simulink subsystem "SurfEngRef"  (R2025a)
settings: Solver=VariableStepAuto  StartTime=0.0  StopTime=10.0  RelTol=1e-3
undefined symbols (not defined in the file): SimIn, SimPar
libraries: simulink x42, ServosLib x6
(part 1 of 2)
settings Model: Creator=drhill  LastModifiedBy=alhallmark
settings SolverCC: AlgebraicLoopSolver=TrustRegion
settings OptimizationCC: ReuseModelBlockBuffer=off
settings DebuggingCC: UnconnectedInputMsg=warning  UnconnectedOutputMsg=warning  UnconnectedLineMsg=warning
settings ModelReferenceCC: EnableRefExpFcnMdlSchedulingChecks=on
settings RTWCC: GPUComputeCapability=3.5  DLArmComputeVersion=19.05

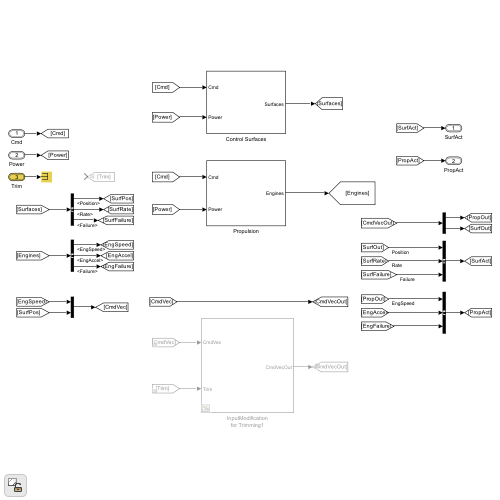
[thumbnail: Simulink's stored preview of the top-level diagram]
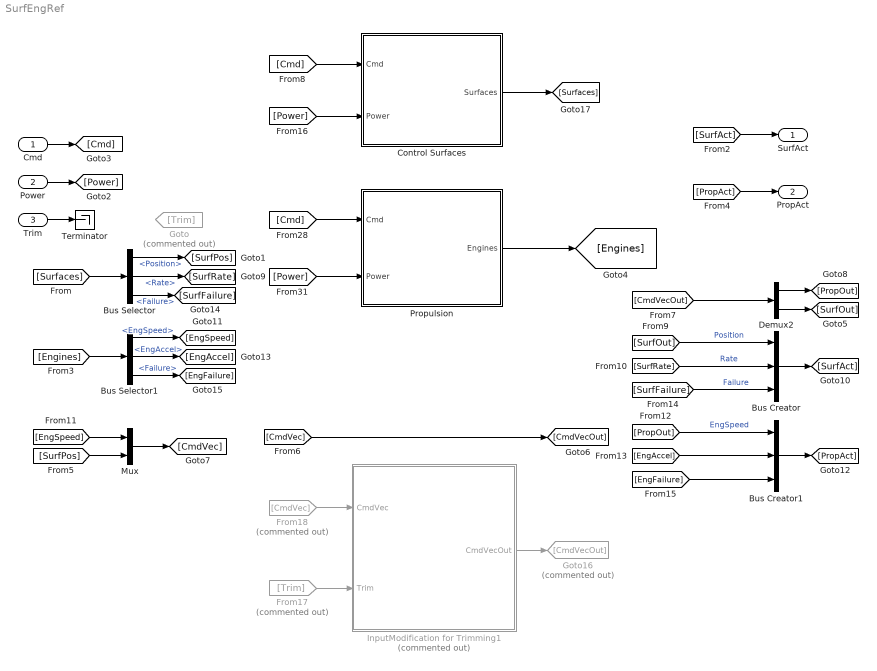
== system SurfEngRef ==
  Cmd : Inport  OutDataTypeStr=Bus: BUS_CMD
  Power : Inport  Port=2  OutDataTypeStr=Bus: BUS_POWER_SYSTEM_OUT
  Trim : Inport  Port=3  OutDataTypeStr=Bus: BUS_TRIM_INPUT
  Bus Creator : BusCreator  Inputs=3  OutDataTypeStr=Bus: BUS_SURF_ACTUATOR
  Bus Creator1 : BusCreator  Inputs=3  OutDataTypeStr=Bus: BUS_PROP_ACTUATOR
  Bus Selector : BusSelector  OutputSignals=Position,Rate,Failure
  Bus Selector1 : BusSelector  OutputSignals=EngSpeed,EngAccel,Failure
  Control Surfaces : Subsystem  VariantControl=GVS_ACT_TYPE_NONE
  Demux2 : Demux  Outputs=[SimIn.numEngines SimIn.numSurfaces]
  From17 : From  Commented=on  GotoTag=Trim
  From18 : From  Commented=on  GotoTag=CmdVec
  Goto : Goto  Commented=on  GotoTag=Trim
  Goto16 : Goto  Commented=on  GotoTag=CmdVecOut
  InputModification for Trimming1 : Subsystem  Commented=on
  Mux : Mux  Inputs=[SimIn.numEngines SimIn.numSurfaces]
  Propulsion : Subsystem  VariantControl=GVS_PROP_TYPE_NONE
  Terminator : Terminator
  SurfAct : Outport  OutDataTypeStr=Bus: BUS_SURF_ACTUATOR
  PropAct : Outport  Port=2  OutDataTypeStr=Bus: BUS_PROP_ACTUATOR
  wires:
  [Cmd] -> Control Surfaces/1(Cmd)
  [Power] -> Control Surfaces/2(Power)
  Control Surfaces/1(Surfaces) -> [Surfaces]
  Trim/1 -> Terminator/1
  Power/1 -> [Power]
  Cmd/1 -> [Cmd]
  [SurfAct] -> SurfAct/1
  [Power] -> Propulsion/2(Power)
  Propulsion/1(Engines) -> [Engines]
  [PropAct] -> PropAct/1
  [Cmd] -> Propulsion/1(Cmd)
  [CmdVec] -> [CmdVecOut]
  Mux/1 -> [CmdVec]
  [CmdVecOut] -> Demux2/1
  Demux2/2 -> [SurfOut]
  Demux2/1 -> [PropOut]
  [Surfaces] -> Bus Selector/1
  Bus Selector/1 -> [SurfPos]  "<Position>"
  [SurfPos] -> Mux/2
  [SurfOut] -> Bus Creator/1  "Position"
  Bus Selector/2 -> [SurfRate]  "<Rate>"
  [SurfRate] -> Bus Creator/2  "Rate"
  Bus Creator/1 -> [SurfAct]
  [Engines] -> Bus Selector1/1
  Bus Selector1/1 -> [EngSpeed]  "<EngSpeed>"
  [EngSpeed] -> Mux/1
  [PropOut] -> Bus Creator1/1  "EngSpeed"
  Bus Creator1/1 -> [PropAct]
  Bus Selector1/2 -> [EngAccel]  "<EngAccel>"
  [EngAccel] -> Bus Creator1/2
  Bus Selector/3 -> [SurfFailure]  "<Failure>"
  [SurfFailure] -> Bus Creator/3  "Failure"
  Bus Selector1/3 -> [EngFailure]  "<Failure>"
  [EngFailure] -> Bus Creator1/3
  InputModification for Trimming1/1(CmdVecOut) -> Goto16/1
  From18/1 -> InputModification for Trimming1/1(CmdVec)
  From17/1 -> InputModification for Trimming1/2(Trim)

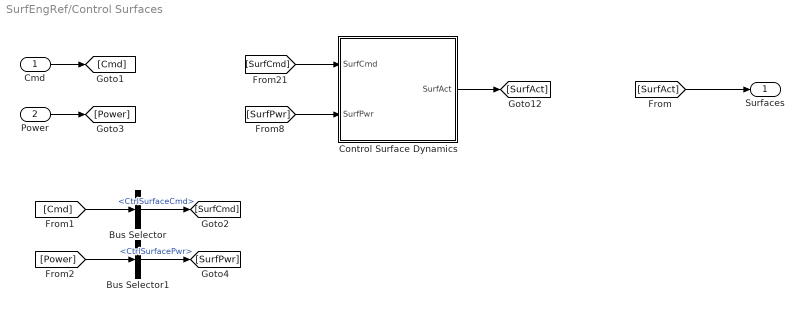
== system SurfEngRef/Control Surfaces ==
  Cmd : Inport
  Power : Inport  Port=2
  Bus Selector : BusSelector  OutputSignals=CtrlSurfaceCmd
  Bus Selector1 : BusSelector  OutputSignals=CtrlSurfacePwr
  Control Surface Dynamics : Subsystem  Variant=on
  Surfaces : Outport  VectorParamsAs1DForOutWhenUnconnected=off
  wires:
  [Cmd] -> Bus Selector/1
  Bus Selector/1 -> [SurfCmd]  "<CtrlSurfaceCmd>"
  Bus Selector1/1 -> [SurfPwr]  "<CtrlSurfacePwr>"
  [Power] -> Bus Selector1/1
  [SurfPwr] -> Control Surface Dynamics/2(SurfPwr)
  Control Surface Dynamics/1(SurfAct) -> [SurfAct]
  [SurfCmd] -> Control Surface Dynamics/1(SurfCmd)
  Power/1 -> [Power]
  [SurfAct] -> Surfaces/1
  Cmd/1 -> [Cmd]

== system SurfEngRef/InputModification for Trimming1 ==
  CmdVec : Inport
  Trim : Inport  Port=2  OutDataTypeStr=Bus: BUS_TRIM_INPUT
  Constant : Constant  Value=SimIn.Switches.TrimModeOn
  "Invalid, Error Out" : Subsystem  TreatAsAtomicUnit=on
  Merge : Merge  Inputs=3  InitialOutput=zeros(SimIn.numEngines+SimIn.numSurfaces,1)
  SimMode:PassThrough : Subsystem  TreatAsAtomicUnit=on
  Switch Case : SwitchCase  CaseConditions={0,1}
  TrimMode: DriveFromTopLevel : Subsystem  TreatAsAtomicUnit=on
  CmdVecOut : Outport  VectorParamsAs1DForOutWhenUnconnected=off
  wires:
  [Trim] -> TrimMode: DriveFromTopLevel/1(TrimBias)
  [CmdVec] -> SimMode:PassThrough/1(Cmd)
  Trim/1 -> [Trim]
  CmdVec/1 -> [CmdVec]
  Switch Case/1 -> SimMode:PassThrough/Action
  Switch Case/2 -> TrimMode: DriveFromTopLevel/Action
  SimMode:PassThrough/1(Out) -> Merge/1
  TrimMode: DriveFromTopLevel/1(Out) -> Merge/2
  Merge/1 -> CmdVecOut/1
  Constant/1 -> Switch Case/1
  Switch Case/3 -> "Invalid, Error Out"/Action
  "Invalid, Error Out"/1(Out) -> Merge/3

== system SurfEngRef/Propulsion ==
  Cmd : Inport  OutDataTypeStr=Bus: BUS_CMD
  Power : Inport  Port=2
  Bus Selector : BusSelector  OutputSignals=EngineCmd
  Bus Selector1 : BusSelector  OutputSignals=EnginePwr
  Propulsion Dynamics : Subsystem  Variant=on
  Engines : Outport  OutDataTypeStr=Bus: BUS_PROP_ACTUATOR  VectorParamsAs1DForOutWhenUnconnected=off
  wires:
  Bus Selector1/1 -> [EngPwr]  "<EnginePwr>"
  [Power] -> Bus Selector1/1
  Bus Selector/1 -> [EngCmd]  "<EngineCmd>"
  [Cmd] -> Bus Selector/1
  [EngPwr] -> Propulsion Dynamics/2(EngPwr)
  [EngCmd] -> Propulsion Dynamics/1(EngCmd)
  Propulsion Dynamics/1(PropAct) -> [PropAct]
  [PropAct] -> Engines/1
  Power/1 -> [Power]
  Cmd/1 -> [Cmd]

== system SurfEngRef/Control Surfaces/Control Surface Dynamics ==
  SurfCmd : Inport
  SurfPwr : Inport  Port=2
  FirstOrder : Subsystem  VariantControl=GVS_ACT_TYPE_FIRSTORDER
  FirstOrderFailSurf : Subsystem  VariantControl=GVS_ACT_TYPE_FIRSTORDERFAILSURF
  None : Subsystem  VariantControl=GVS_ACT_TYPE_NONE
  SecondOrder : Subsystem  VariantControl=GVS_ACT_TYPE_SECONDORDER
  SurfAct : Outport

== system SurfEngRef/InputModification for Trimming1/Invalid, Error Out ==
  Action Port : ActionPort
  Constant1 : Constant  Value=zeros(SimIn.numEngines+SimIn.numSurfaces,1)
  Constant2 : Constant  Value=0
  InvalidMode : Assertion  AssertionFailFcn="warndlg('Invalid settings for TrimMode and LinearizeMode.  Run setup.m to reset.','Warning!')"
  Out : Outport  InitialOutput=zeros(SimIn.numEngines+SimIn.numSurfaces,1)  VectorParamsAs1DForOutWhenUnconnected=off
  wires:
  Constant2/1 -> InvalidMode/1
  Constant1/1 -> Out/1

== system SurfEngRef/InputModification for Trimming1/SimMode:PassThrough ==
  Cmd : Inport
  Action Port : ActionPort
  Gain1 : Gain
  Out : Outport  InitialOutput=zeros(SimIn.numEngines+SimIn.numSurfaces,1)  VectorParamsAs1DForOutWhenUnconnected=off
  wires:
  Cmd/1 -> Gain1/1  "LiftEngines(8),TailEngine,Aileron,Flaps,Elevator,Rudder"
  Gain1/1 -> Out/1

== system SurfEngRef/InputModification for Trimming1/TrimMode: DriveFromTopLevel ==
  TrimBias : Inport  OutDataTypeStr=Bus: BUS_TRIM_INPUT
  Action Port : ActionPort
  Bus Selector : BusSelector  OutputSignals=Engines,Surfaces
  Force Consistent Sample Time on Bus : Subsystem  Commented=on
  Multiply : Gain  Gain=SimIn.Trim.surfaceAlloc  Multiplication=Matrix(K*u)
  Mux : Mux  Inputs=2
  Out : Outport  InitialOutput=zeros(SimIn.numEngines+SimIn.numSurfaces,1)  VectorParamsAs1DForOutWhenUnconnected=off
  wires:
  Mux/1 -> Out/1
  Multiply/1 -> Mux/2
  Bus Selector/1 -> Mux/1  "<Engines>"
  TrimBias/1 -> Bus Selector/1
  Bus Selector/2 -> Multiply/1  "<Surfaces>"

== system SurfEngRef/Propulsion/Propulsion Dynamics ==
  EngCmd : Inport
  EngPwr : Inport  Port=2
  FirstOrder : Subsystem  VariantControl=GVS_PROP_TYPE_FIRSTORDER
  FirstOrderFailProp : Subsystem  VariantControl=GVS_PROP_TYPE_FIRSTORDERFAILPROP
  None : Subsystem  VariantControl=GVS_PROP_TYPE_NONE
  SecondOrder : Subsystem  VariantControl=GVS_PROP_TYPE_SECONDORDER
  PropAct : Outport

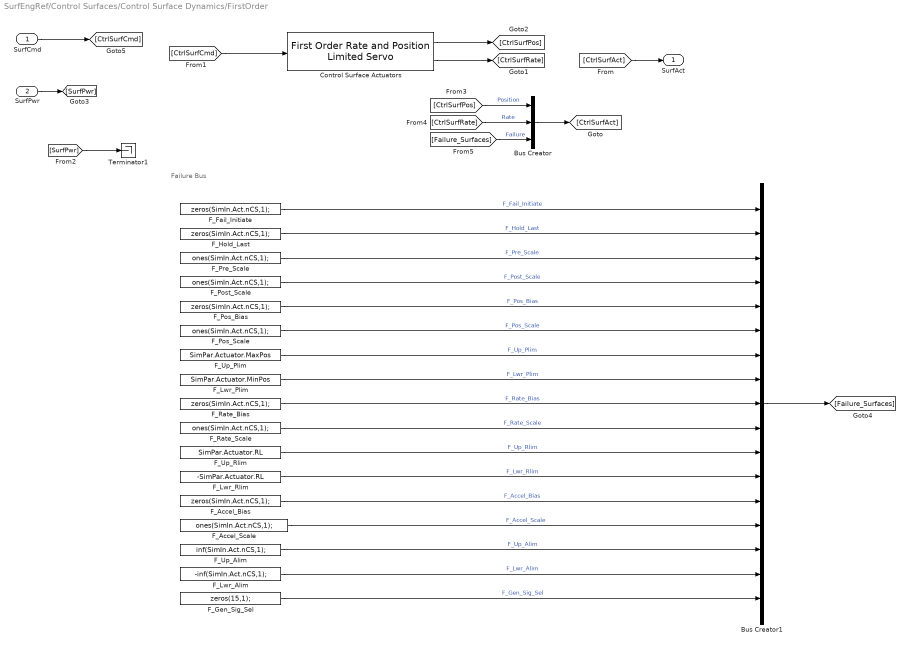
== system SurfEngRef/Control Surfaces/Control Surface Dynamics/FirstOrder ==
  note: Failure Bus
  SurfCmd : Inport
  SurfPwr : Inport  Port=2
  Bus Creator : BusCreator  Inputs=3  OutDataTypeStr=Bus: BUS_SURF_ACTUATOR
  Bus Creator1 : BusCreator  Inputs=17  OutDataTypeStr=Bus: BUS_FAILURE_SURF
  Control Surface Actuators : ServosLib/First Order  Rate and Position Limited  Servo  freq=SimPar.Actuator.BW  RL=SimPar.Actuator.RL  POS_hi=SimPar.Actuator.MaxPos  POS_lo=SimPar.Actuator.MinPos  Bias=SimPar.Actuator.Bias  StateName=Actuators
  F_Accel_Bias : Constant  Value=zeros(SimIn.Act.nCS,1);
  F_Accel_Scale : Constant  Value=ones(SimIn.Act.nCS,1);
  F_Fail_Initiate : Constant  Value=zeros(SimIn.Act.nCS,1);
  F_Gen_Sig_Sel : Constant  Value=zeros(15,1);
  F_Hold_Last : Constant  Value=zeros(SimIn.Act.nCS,1);
  F_Lwr_Alim : Constant  Value=-inf(SimIn.Act.nCS,1);
  F_Lwr_Plim : Constant  Value=SimPar.Actuator.MinPos
  F_Lwr_Rlim : Constant  Value=-SimPar.Actuator.RL
  F_Pos_Bias : Constant  Value=zeros(SimIn.Act.nCS,1);
  F_Pos_Scale : Constant  Value=ones(SimIn.Act.nCS,1);
  F_Post_Scale : Constant  Value=ones(SimIn.Act.nCS,1);
  F_Pre_Scale : Constant  Value=ones(SimIn.Act.nCS,1);
  F_Rate_Bias : Constant  Value=zeros(SimIn.Act.nCS,1);
  F_Rate_Scale : Constant  Value=ones(SimIn.Act.nCS,1);
  F_Up_Alim : Constant  Value=inf(SimIn.Act.nCS,1);
  F_Up_Plim : Constant  Value=SimPar.Actuator.MaxPos
  F_Up_Rlim : Constant  Value=SimPar.Actuator.RL
  Terminator1 : Terminator
  SurfAct : Outport
  wires:
  F_Gen_Sig_Sel/1 -> Bus Creator1/17  "F_Gen_Sig_Sel"
  F_Lwr_Alim/1 -> Bus Creator1/16  "F_Lwr_Alim"
  F_Up_Alim/1 -> Bus Creator1/15  "F_Up_Alim"
  F_Accel_Scale/1 -> Bus Creator1/14  "F_Accel_Scale"
  F_Accel_Bias/1 -> Bus Creator1/13  "F_Accel_Bias"
  F_Lwr_Rlim/1 -> Bus Creator1/12  "F_Lwr_Rlim"
  F_Up_Rlim/1 -> Bus Creator1/11  "F_Up_Rlim"
  F_Rate_Scale/1 -> Bus Creator1/10  "F_Rate_Scale"
  F_Rate_Bias/1 -> Bus Creator1/9  "F_Rate_Bias"
  F_Lwr_Plim/1 -> Bus Creator1/8  "F_Lwr_Plim"
  F_Up_Plim/1 -> Bus Creator1/7  "F_Up_Plim"
  F_Pos_Scale/1 -> Bus Creator1/6  "F_Pos_Scale"
  F_Pos_Bias/1 -> Bus Creator1/5  "F_Pos_Bias"
  F_Post_Scale/1 -> Bus Creator1/4  "F_Post_Scale"
  [Failure_Surfaces] -> Bus Creator/3  "Failure"
  F_Pre_Scale/1 -> Bus Creator1/3  "F_Pre_Scale"
  F_Hold_Last/1 -> Bus Creator1/2  "F_Hold_Last"
  Bus Creator1/1 -> [Failure_Surfaces]
  F_Fail_Initiate/1 -> Bus Creator1/1  "F_Fail_Initiate"
  [SurfPwr] -> Terminator1/1
  SurfPwr/1 -> [SurfPwr]
  SurfCmd/1 -> [CtrlSurfCmd]
  [CtrlSurfCmd] -> Control Surface Actuators/1
  Control Surface Actuators/1 -> [CtrlSurfPos]
  Control Surface Actuators/2 -> [CtrlSurfRate]
  [CtrlSurfAct] -> SurfAct/1
  [CtrlSurfPos] -> Bus Creator/1  "Position"
  [CtrlSurfRate] -> Bus Creator/2  "Rate"
  Bus Creator/1 -> [CtrlSurfAct]

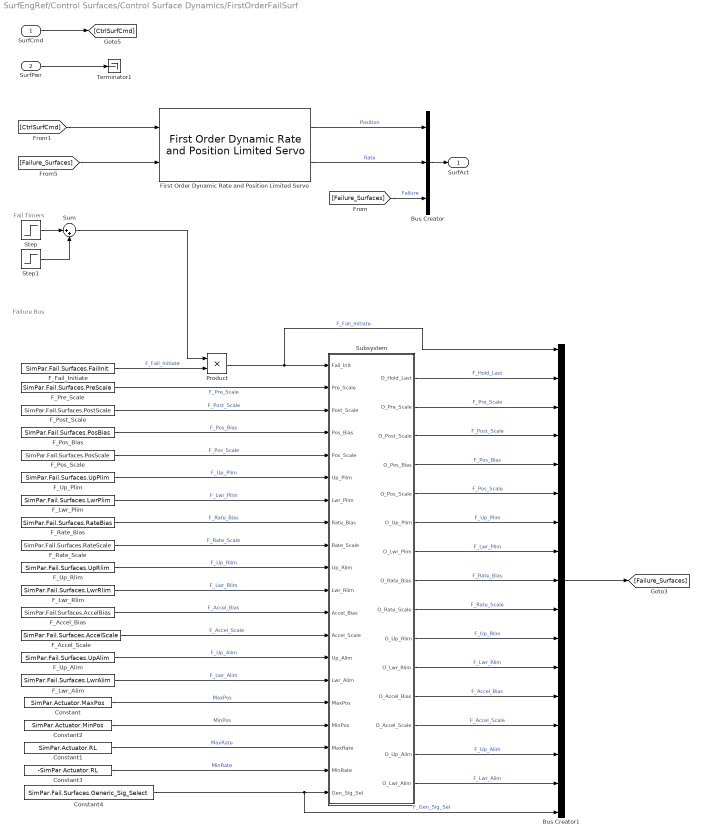
== system SurfEngRef/Control Surfaces/Control Surface Dynamics/FirstOrderFailSurf ==
  note: Failure Bus
  note: Fail Timers
  SurfCmd : Inport
  SurfPwr : Inport  Port=2
  Bus Creator : BusCreator  Inputs=3  OutDataTypeStr=Bus: BUS_SURF_ACTUATOR
  Bus Creator1 : BusCreator  Inputs=17  OutDataTypeStr=Bus: BUS_FAILURE_SURF
  Constant : Constant  Value=SimPar.Actuator.MaxPos
  Constant1 : Constant  Value=SimPar.Actuator.RL
  Constant2 : Constant  Value=SimPar.Actuator.MinPos
  Constant3 : Constant  Value=-SimPar.Actuator.RL
  Constant4 : Constant  Value=SimPar.Fail.Surfaces.Generic_Sig_Select
  F_Accel_Bias : Constant  Value=SimPar.Fail.Surfaces.AccelBias
  F_Accel_Scale : Constant  Value=SimPar.Fail.Surfaces.AccelScale
  F_Fail_Initiate : Constant  Value=SimPar.Fail.Surfaces.FailInit
  F_Lwr_Alim : Constant  Value=SimPar.Fail.Surfaces.LwrAlim
  F_Lwr_Plim : Constant  Value=SimPar.Fail.Surfaces.LwrPlim
  F_Lwr_Rlim : Constant  Value=SimPar.Fail.Surfaces.LwrRlim
  F_Pos_Bias : Constant  Value=SimPar.Fail.Surfaces.PosBias
  F_Pos_Scale : Constant  Value=SimPar.Fail.Surfaces.PosScale
  F_Post_Scale : Constant  Value=SimPar.Fail.Surfaces.PostScale
  F_Pre_Scale : Constant  Value=SimPar.Fail.Surfaces.PreScale
  F_Rate_Bias : Constant  Value=SimPar.Fail.Surfaces.RateBias
  F_Rate_Scale : Constant  Value=SimPar.Fail.Surfaces.RateScale
  F_Up_Alim : Constant  Value=SimPar.Fail.Surfaces.UpAlim
  F_Up_Plim : Constant  Value=SimPar.Fail.Surfaces.UpPlim
  F_Up_Rlim : Constant  Value=SimPar.Fail.Surfaces.UpRlim
  First Order Dynamic Rate and Position Limited Servo : ServosLib/First Order Dynamic Rate and Position Limited Servo  freq=SimPar.Actuator.BW  Bias=SimPar.Actuator.Bias  StateName='Actuators'
  Product : Product
  Step : Step  Time=SimPar.Fail.Surfaces.InitTime  SampleTime=0
  Step1 : Step  Time=SimPar.Fail.Surfaces.StopTime  After=-1  SampleTime=0
  Subsystem : Subsystem
  Sum : Sum  Inputs=|++
  Terminator1 : Terminator
  SurfAct : Outport
  wires:
  [Failure_Surfaces] -> Bus Creator/3  "Failure"
  Constant4/1 -> Bus Creator1/17, Subsystem/20(Gen_Sig_Sel)  "F_Gen_Sig_Sel"
  Sum/1 -> Product/1
  Product/1 -> Subsystem/1(Fail_Init), Bus Creator1/1  "F_Fail_Initiate"
  Step1/1 -> Sum/2
  Step/1 -> Sum/1
  Subsystem/13(O_Accel_Scale) -> Bus Creator1/14  "F_Accel_Scale"
  Subsystem/12(O_Accel_Bias) -> Bus Creator1/13  "F_Accel_Bias"
  Subsystem/15(O_Lwr_Alim) -> Bus Creator1/16  "F_Lwr_Alim"
  Subsystem/14(O_Up_Alim) -> Bus Creator1/15  "F_Up_Alim"
  Subsystem/11(O_Lwr_Rlim) -> Bus Creator1/12  "F_Lwr_Rlim"
  Subsystem/10(O_Up_Rlim) -> Bus Creator1/11  "F_Up_Rlim"
  Subsystem/9(O_Rate_Scale) -> Bus Creator1/10  "F_Rate_Scale"
  Subsystem/8(O_Rate_Bias) -> Bus Creator1/9  "F_Rate_Bias"
  Subsystem/7(O_Lwr_Plim) -> Bus Creator1/8  "F_Lwr_Plim"
  Subsystem/6(O_Up_Plim) -> Bus Creator1/7  "F_Up_Plim"
  Subsystem/5(O_Pos_Scale) -> Bus Creator1/6  "F_Pos_Scale"
  Subsystem/4(O_Pos_Bias) -> Bus Creator1/5  "F_Pos_Bias"
  Subsystem/3(O_Post_Scale) -> Bus Creator1/4  "F_Post_Scale"
  Subsystem/2(O_Pre_Scale) -> Bus Creator1/3  "F_Pre_Scale"
  Subsystem/1(O_Hold_Last) -> Bus Creator1/2  "F_Hold_Last"
  Bus Creator1/1 -> [Failure_Surfaces]
  F_Post_Scale/1 -> Subsystem/3(Post_Scale)  "F_Post_Scale"
  F_Accel_Scale/1 -> Subsystem/13(Accel_Scale)  "F_Accel_Scale"
  F_Lwr_Alim/1 -> Subsystem/15(Lwr_Alim)  "F_Lwr_Alim"
  [Failure_Surfaces] -> First Order Dynamic Rate and Position Limited Servo/2
  [CtrlSurfCmd] -> First Order Dynamic Rate and Position Limited Servo/1
  First Order Dynamic Rate and Position Limited Servo/2 -> Bus Creator/2  "Rate"
  F_Lwr_Plim/1 -> Subsystem/7(Lwr_Plim)  "F_Lwr_Plim"
  F_Up_Plim/1 -> Subsystem/6(Up_Plim)  "F_Up_Plim"
  F_Pos_Bias/1 -> Subsystem/4(Pos_Bias)  "F_Pos_Bias"
  F_Rate_Bias/1 -> Subsystem/8(Rate_Bias)  "F_Rate_Bias"
  F_Lwr_Rlim/1 -> Subsystem/11(Lwr_Rlim)  "F_Lwr_Rlim"
  F_Fail_Initiate/1 -> Product/2  "F_Fail_Initiate"
  SurfPwr/1 -> Terminator1/1
  Constant1/1 -> Subsystem/18(MaxRate)  "MaxRate"
  Constant3/1 -> Subsystem/19(MinRate)  "MinRate"
  F_Pos_Scale/1 -> Subsystem/5(Pos_Scale)  "F_Pos_Scale"
  Bus Creator/1 -> SurfAct/1
  Constant2/1 -> Subsystem/17(MinPos)  "MinPos"
  Constant/1 -> Subsystem/16(MaxPos)  "MaxPos"
  F_Pre_Scale/1 -> Subsystem/2(Pre_Scale)  "F_Pre_Scale"
  F_Up_Alim/1 -> Subsystem/14(Up_Alim)  "F_Up_Alim"
  F_Rate_Scale/1 -> Subsystem/9(Rate_Scale)  "F_Rate_Scale"
  F_Accel_Bias/1 -> Subsystem/12(Accel_Bias)  "F_Accel_Bias"
  SurfCmd/1 -> [CtrlSurfCmd]
  F_Up_Rlim/1 -> Subsystem/10(Up_Rlim)  "F_Up_Rlim"
  First Order Dynamic Rate and Position Limited Servo/1 -> Bus Creator/1  "Position"

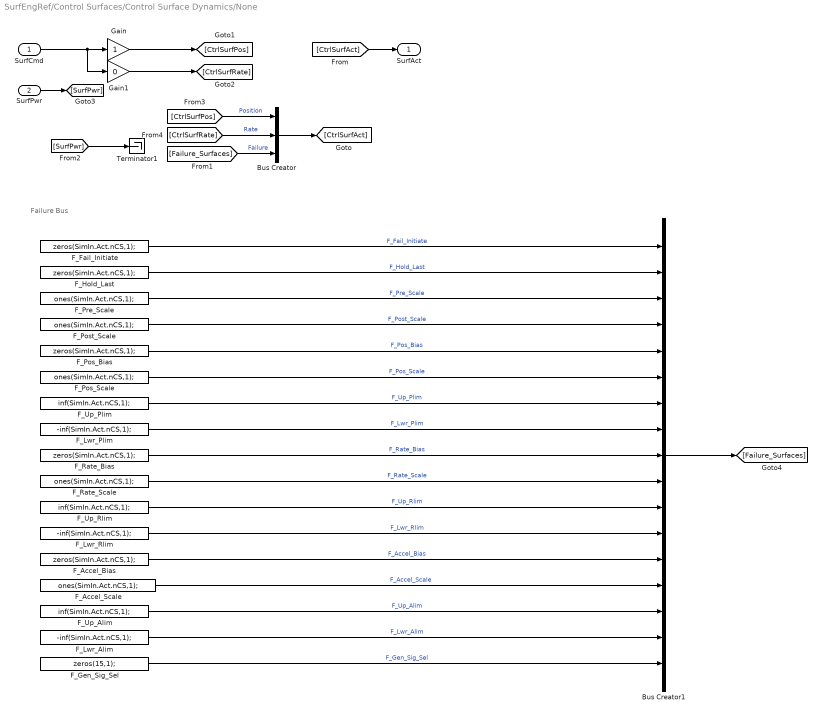
== system SurfEngRef/Control Surfaces/Control Surface Dynamics/None ==
  note: Failure Bus
  SurfCmd : Inport
  SurfPwr : Inport  Port=2
  Bus Creator : BusCreator  Inputs=3  OutDataTypeStr=Bus: BUS_SURF_ACTUATOR
  Bus Creator1 : BusCreator  Inputs=17  OutDataTypeStr=Bus: BUS_FAILURE_SURF
  F_Accel_Bias : Constant  Value=zeros(SimIn.Act.nCS,1);
  F_Accel_Scale : Constant  Value=ones(SimIn.Act.nCS,1);
  F_Fail_Initiate : Constant  Value=zeros(SimIn.Act.nCS,1);
  F_Gen_Sig_Sel : Constant  Value=zeros(15,1);
  F_Hold_Last : Constant  Value=zeros(SimIn.Act.nCS,1);
  F_Lwr_Alim : Constant  Value=-inf(SimIn.Act.nCS,1);
  F_Lwr_Plim : Constant  Value=-inf(SimIn.Act.nCS,1);
  F_Lwr_Rlim : Constant  Value=-inf(SimIn.Act.nCS,1);
  F_Pos_Bias : Constant  Value=zeros(SimIn.Act.nCS,1);
  F_Pos_Scale : Constant  Value=ones(SimIn.Act.nCS,1);
  F_Post_Scale : Constant  Value=ones(SimIn.Act.nCS,1);
  F_Pre_Scale : Constant  Value=ones(SimIn.Act.nCS,1);
  F_Rate_Bias : Constant  Value=zeros(SimIn.Act.nCS,1);
  F_Rate_Scale : Constant  Value=ones(SimIn.Act.nCS,1);
  F_Up_Alim : Constant  Value=inf(SimIn.Act.nCS,1);
  F_Up_Plim : Constant  Value=inf(SimIn.Act.nCS,1);
  F_Up_Rlim : Constant  Value=inf(SimIn.Act.nCS,1);
  Gain : Gain
  Gain1 : Gain  Gain=0
  Terminator1 : Terminator
  SurfAct : Outport
  wires:
  F_Gen_Sig_Sel/1 -> Bus Creator1/17  "F_Gen_Sig_Sel"
  F_Lwr_Alim/1 -> Bus Creator1/16  "F_Lwr_Alim"
  F_Up_Alim/1 -> Bus Creator1/15  "F_Up_Alim"
  F_Accel_Scale/1 -> Bus Creator1/14  "F_Accel_Scale"
  F_Accel_Bias/1 -> Bus Creator1/13  "F_Accel_Bias"
  F_Lwr_Rlim/1 -> Bus Creator1/12  "F_Lwr_Rlim"
  F_Up_Rlim/1 -> Bus Creator1/11  "F_Up_Rlim"
  F_Rate_Scale/1 -> Bus Creator1/10  "F_Rate_Scale"
  F_Rate_Bias/1 -> Bus Creator1/9  "F_Rate_Bias"
  F_Lwr_Plim/1 -> Bus Creator1/8  "F_Lwr_Plim"
  F_Up_Plim/1 -> Bus Creator1/7  "F_Up_Plim"
  F_Pos_Scale/1 -> Bus Creator1/6  "F_Pos_Scale"
  F_Pos_Bias/1 -> Bus Creator1/5  "F_Pos_Bias"
  F_Post_Scale/1 -> Bus Creator1/4  "F_Post_Scale"
  F_Pre_Scale/1 -> Bus Creator1/3  "F_Pre_Scale"
  [Failure_Surfaces] -> Bus Creator/3  "Failure"
  F_Fail_Initiate/1 -> Bus Creator1/1  "F_Fail_Initiate"
  Bus Creator1/1 -> [Failure_Surfaces]
  F_Hold_Last/1 -> Bus Creator1/2  "F_Hold_Last"
  Gain1/1 -> [CtrlSurfRate]
  Gain/1 -> [CtrlSurfPos]
  [CtrlSurfAct] -> SurfAct/1
  [CtrlSurfRate] -> Bus Creator/2  "Rate"
  [CtrlSurfPos] -> Bus Creator/1  "Position"
  Bus Creator/1 -> [CtrlSurfAct]
  [SurfPwr] -> Terminator1/1
  SurfPwr/1 -> [SurfPwr]
  SurfCmd/1 -> Gain1/1, Gain/1

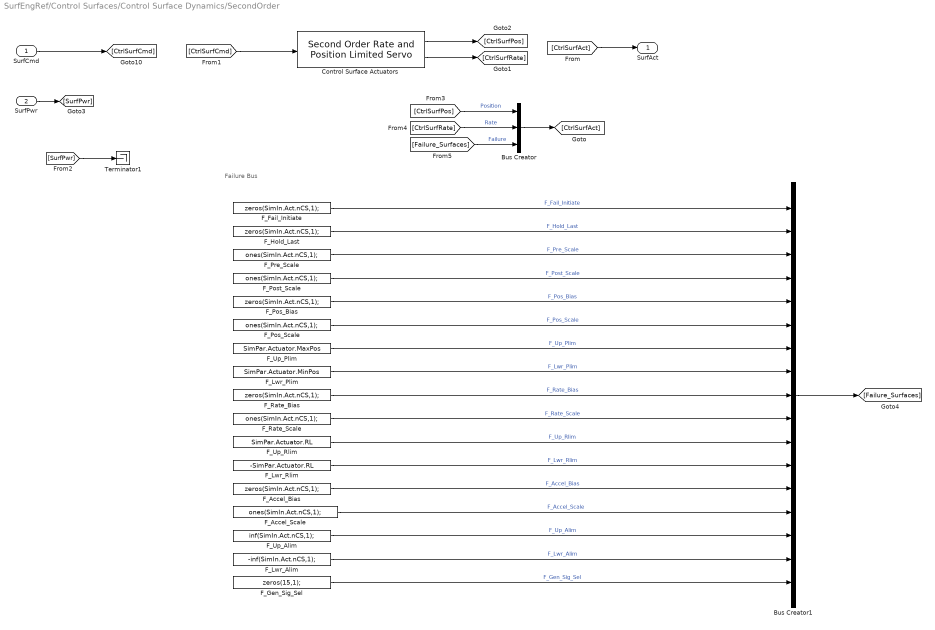
== system SurfEngRef/Control Surfaces/Control Surface Dynamics/SecondOrder ==
  note: Failure Bus
  SurfCmd : Inport
  SurfPwr : Inport  Port=2
  Bus Creator : BusCreator  Inputs=3  OutDataTypeStr=Bus: BUS_SURF_ACTUATOR
  Bus Creator1 : BusCreator  Inputs=17  OutDataTypeStr=Bus: BUS_FAILURE_SURF
  Control Surface Actuators : ServosLib/Second Order Rate and Position Limited Servo  freq=SimPar.Actuator.BW  zeta=SimPar.Actuator.Zeta  RL=SimPar.Actuator.RL  POS_hi=SimPar.Actuator.MaxPos  POS_lo=SimPar.Actuator.MinPos  Bias=SimPar.Actuator.Bias  PosStateName=ActuatorPosition  RateStateName=ActuatorRate
  F_Accel_Bias : Constant  Value=zeros(SimIn.Act.nCS,1);
  F_Accel_Scale : Constant  Value=ones(SimIn.Act.nCS,1);
  F_Fail_Initiate : Constant  Value=zeros(SimIn.Act.nCS,1);
  F_Gen_Sig_Sel : Constant  Value=zeros(15,1);
  F_Hold_Last : Constant  Value=zeros(SimIn.Act.nCS,1);
  F_Lwr_Alim : Constant  Value=-inf(SimIn.Act.nCS,1);
  F_Lwr_Plim : Constant  Value=SimPar.Actuator.MinPos
  F_Lwr_Rlim : Constant  Value=-SimPar.Actuator.RL
  F_Pos_Bias : Constant  Value=zeros(SimIn.Act.nCS,1);
  F_Pos_Scale : Constant  Value=ones(SimIn.Act.nCS,1);
  F_Post_Scale : Constant  Value=ones(SimIn.Act.nCS,1);
  F_Pre_Scale : Constant  Value=ones(SimIn.Act.nCS,1);
  F_Rate_Bias : Constant  Value=zeros(SimIn.Act.nCS,1);
  F_Rate_Scale : Constant  Value=ones(SimIn.Act.nCS,1);
  F_Up_Alim : Constant  Value=inf(SimIn.Act.nCS,1);
  F_Up_Plim : Constant  Value=SimPar.Actuator.MaxPos
  F_Up_Rlim : Constant  Value=SimPar.Actuator.RL
  Terminator1 : Terminator
  SurfAct : Outport
  wires:
  F_Lwr_Alim/1 -> Bus Creator1/16  "F_Lwr_Alim"
  F_Rate_Scale/1 -> Bus Creator1/10  "F_Rate_Scale"
  F_Rate_Bias/1 -> Bus Creator1/9  "F_Rate_Bias"
  F_Post_Scale/1 -> Bus Creator1/4  "F_Post_Scale"
  F_Up_Rlim/1 -> Bus Creator1/11  "F_Up_Rlim"
  F_Lwr_Rlim/1 -> Bus Creator1/12  "F_Lwr_Rlim"
  F_Hold_Last/1 -> Bus Creator1/2  "F_Hold_Last"
  F_Lwr_Plim/1 -> Bus Creator1/8  "F_Lwr_Plim"
  F_Accel_Bias/1 -> Bus Creator1/13  "F_Accel_Bias"
  F_Gen_Sig_Sel/1 -> Bus Creator1/17  "F_Gen_Sig_Sel"
  F_Accel_Scale/1 -> Bus Creator1/14  "F_Accel_Scale"
  F_Up_Alim/1 -> Bus Creator1/15  "F_Up_Alim"
  F_Pre_Scale/1 -> Bus Creator1/3  "F_Pre_Scale"
  F_Up_Plim/1 -> Bus Creator1/7  "F_Up_Plim"
  F_Pos_Bias/1 -> Bus Creator1/5  "F_Pos_Bias"
  F_Pos_Scale/1 -> Bus Creator1/6  "F_Pos_Scale"
  F_Fail_Initiate/1 -> Bus Creator1/1  "F_Fail_Initiate"
  Bus Creator1/1 -> [Failure_Surfaces]
  [Failure_Surfaces] -> Bus Creator/3  "Failure"
  [CtrlSurfRate] -> Bus Creator/2  "Rate"
  [CtrlSurfPos] -> Bus Creator/1  "Position"
  Bus Creator/1 -> [CtrlSurfAct]
  Control Surface Actuators/2 -> [CtrlSurfRate]
  Control Surface Actuators/1 -> [CtrlSurfPos]
  [SurfPwr] -> Terminator1/1
  SurfCmd/1 -> [CtrlSurfCmd]
  [CtrlSurfCmd] -> Control Surface Actuators/1
  [CtrlSurfAct] -> SurfAct/1
  SurfPwr/1 -> [SurfPwr]

== system SurfEngRef/InputModification for Trimming1/TrimMode: DriveFromTopLevel/Force Consistent Sample Time on Bus ==
  TrimBias : Inport
  Bus to Vector : BusToVector
  Map4 : Gain
  Out1 : Outport  VectorParamsAs1DForOutWhenUnconnected=off
  wires:
  Bus to Vector/1 -> Map4/1
  Map4/1 -> Out1/1
  TrimBias/1 -> Bus to Vector/1

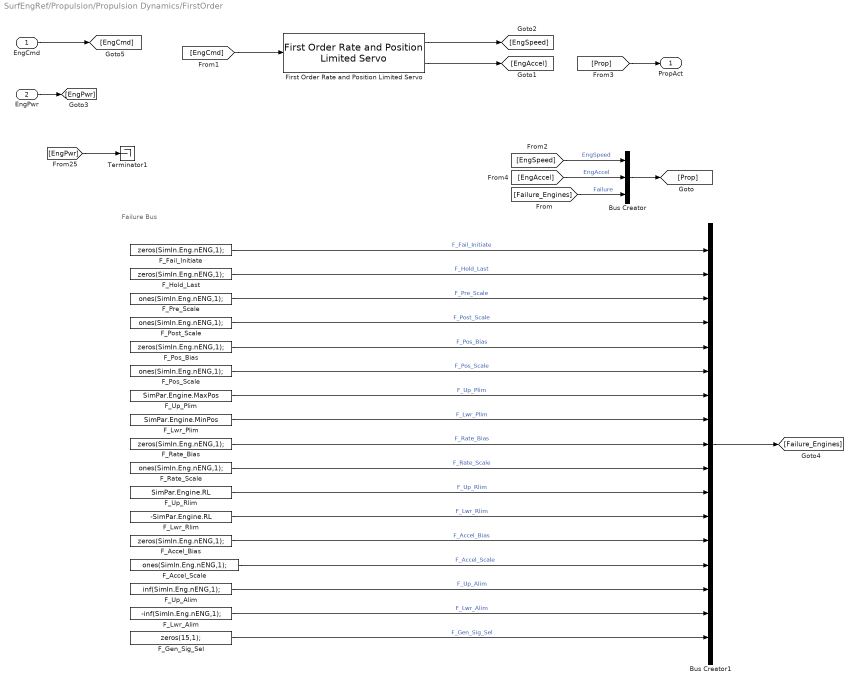
== system SurfEngRef/Propulsion/Propulsion Dynamics/FirstOrder ==
  note: Failure Bus
  EngCmd : Inport
  EngPwr : Inport  Port=2
  Bus Creator : BusCreator  Inputs=3  OutDataTypeStr=Bus: BUS_PROP_ACTUATOR
  Bus Creator1 : BusCreator  Inputs=17  OutDataTypeStr=Bus: BUS_FAILURE_ENG
  F_Accel_Bias : Constant  Value=zeros(SimIn.Eng.nENG,1);
  F_Accel_Scale : Constant  Value=ones(SimIn.Eng.nENG,1);
  F_Fail_Initiate : Constant  Value=zeros(SimIn.Eng.nENG,1);
  F_Gen_Sig_Sel : Constant  Value=zeros(15,1);
  F_Hold_Last : Constant  Value=zeros(SimIn.Eng.nENG,1);
  F_Lwr_Alim : Constant  Value=-inf(SimIn.Eng.nENG,1);
  F_Lwr_Plim : Constant  Value=SimPar.Engine.MinPos
  F_Lwr_Rlim : Constant  Value=-SimPar.Engine.RL
  F_Pos_Bias : Constant  Value=zeros(SimIn.Eng.nENG,1);
  F_Pos_Scale : Constant  Value=ones(SimIn.Eng.nENG,1);
  F_Post_Scale : Constant  Value=ones(SimIn.Eng.nENG,1);
  F_Pre_Scale : Constant  Value=ones(SimIn.Eng.nENG,1);
  F_Rate_Bias : Constant  Value=zeros(SimIn.Eng.nENG,1);
  F_Rate_Scale : Constant  Value=ones(SimIn.Eng.nENG,1);
  F_Up_Alim : Constant  Value=inf(SimIn.Eng.nENG,1);
  F_Up_Plim : Constant  Value=SimPar.Engine.MaxPos
  F_Up_Rlim : Constant  Value=SimPar.Engine.RL
  First Order Rate and Position Limited Servo : ServosLib/First Order  Rate and Position Limited  Servo  freq=SimPar.Engine.BW  RL=SimPar.Engine.RL  POS_hi=SimPar.Engine.MaxPos  POS_lo=SimPar.Engine.MinPos  Bias=SimPar.Engine.Bias  StateName=EngineSpeed
  Terminator1 : Terminator
  PropAct : Outport
  wires:
  [Failure_Engines] -> Bus Creator/3  "Failure"
  F_Lwr_Alim/1 -> Bus Creator1/16  "F_Lwr_Alim"
  F_Rate_Scale/1 -> Bus Creator1/10  "F_Rate_Scale"
  F_Rate_Bias/1 -> Bus Creator1/9  "F_Rate_Bias"
  F_Post_Scale/1 -> Bus Creator1/4  "F_Post_Scale"
  F_Up_Rlim/1 -> Bus Creator1/11  "F_Up_Rlim"
  F_Lwr_Rlim/1 -> Bus Creator1/12  "F_Lwr_Rlim"
  F_Hold_Last/1 -> Bus Creator1/2  "F_Hold_Last"
  F_Lwr_Plim/1 -> Bus Creator1/8  "F_Lwr_Plim"
  F_Accel_Bias/1 -> Bus Creator1/13  "F_Accel_Bias"
  F_Gen_Sig_Sel/1 -> Bus Creator1/17  "F_Gen_Sig_Sel"
  F_Accel_Scale/1 -> Bus Creator1/14  "F_Accel_Scale"
  F_Up_Alim/1 -> Bus Creator1/15  "F_Up_Alim"
  F_Pre_Scale/1 -> Bus Creator1/3  "F_Pre_Scale"
  F_Up_Plim/1 -> Bus Creator1/7  "F_Up_Plim"
  F_Pos_Bias/1 -> Bus Creator1/5  "F_Pos_Bias"
  F_Pos_Scale/1 -> Bus Creator1/6  "F_Pos_Scale"
  F_Fail_Initiate/1 -> Bus Creator1/1  "F_Fail_Initiate"
  Bus Creator1/1 -> [Failure_Engines]
  First Order Rate and Position Limited Servo/2 -> [EngAccel]
  First Order Rate and Position Limited Servo/1 -> [EngSpeed]
  [Prop] -> PropAct/1
  [EngPwr] -> Terminator1/1
  [EngCmd] -> First Order Rate and Position Limited Servo/1
  EngPwr/1 -> [EngPwr]
  EngCmd/1 -> [EngCmd]
  [EngSpeed] -> Bus Creator/1  "EngSpeed"
  Bus Creator/1 -> [Prop]
  [EngAccel] -> Bus Creator/2  "EngAccel"

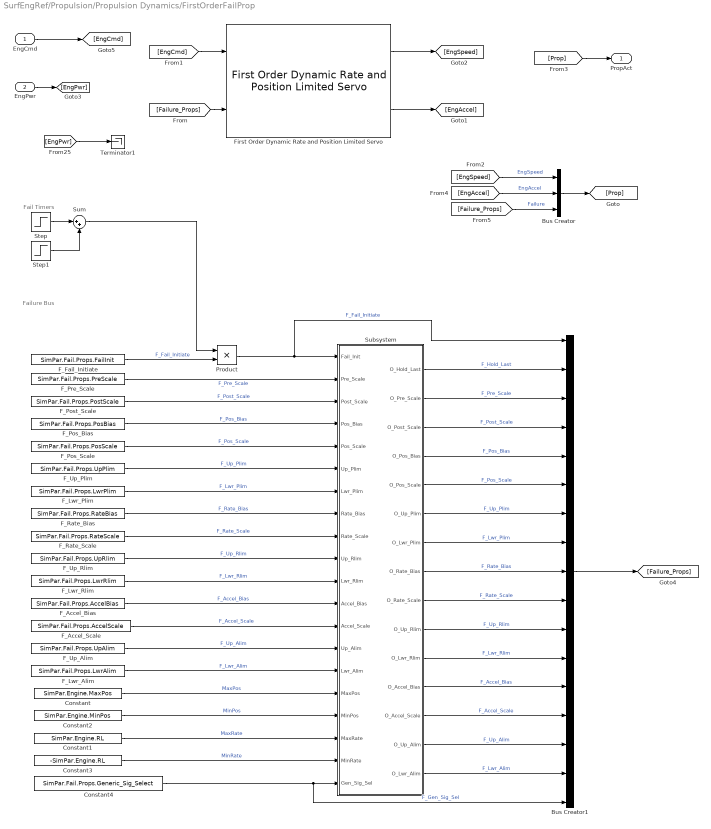
== system SurfEngRef/Propulsion/Propulsion Dynamics/FirstOrderFailProp ==
  note: Failure Bus
  note: Fail Timers
  EngCmd : Inport
  EngPwr : Inport  Port=2
  Bus Creator : BusCreator  Inputs=3  OutDataTypeStr=Bus: BUS_PROP_ACTUATOR
  Bus Creator1 : BusCreator  Inputs=17  OutDataTypeStr=Bus: BUS_FAILURE_ENG
  Constant : Constant  Value=SimPar.Engine.MaxPos
  Constant1 : Constant  Value=SimPar.Engine.RL
  Constant2 : Constant  Value=SimPar.Engine.MinPos
  Constant3 : Constant  Value=-SimPar.Engine.RL
  Constant4 : Constant  Value=SimPar.Fail.Props.Generic_Sig_Select
  F_Accel_Bias : Constant  Value=SimPar.Fail.Props.AccelBias
  F_Accel_Scale : Constant  Value=SimPar.Fail.Props.AccelScale
  F_Fail_Initiate : Constant  Value=SimPar.Fail.Props.FailInit
  F_Lwr_Alim : Constant  Value=SimPar.Fail.Props.LwrAlim
  F_Lwr_Plim : Constant  Value=SimPar.Fail.Props.LwrPlim
  F_Lwr_Rlim : Constant  Value=SimPar.Fail.Props.LwrRlim
  F_Pos_Bias : Constant  Value=SimPar.Fail.Props.PosBias
  F_Pos_Scale : Constant  Value=SimPar.Fail.Props.PosScale
  F_Post_Scale : Constant  Value=SimPar.Fail.Props.PostScale
  F_Pre_Scale : Constant  Value=SimPar.Fail.Props.PreScale
  F_Rate_Bias : Constant  Value=SimPar.Fail.Props.RateBias
  F_Rate_Scale : Constant  Value=SimPar.Fail.Props.RateScale
  F_Up_Alim : Constant  Value=SimPar.Fail.Props.UpAlim
  F_Up_Plim : Constant  Value=SimPar.Fail.Props.UpPlim
  F_Up_Rlim : Constant  Value=SimPar.Fail.Props.UpRlim
  First Order Dynamic Rate and Position Limited Servo : ServosLib/First Order Dynamic Rate and Position Limited Servo  freq=SimPar.Engine.BW  Bias=SimPar.Engine.Bias  StateName='Engines'
  Product : Product
  Step : Step  Time=SimPar.Fail.Props.InitTime  SampleTime=0
  Step1 : Step  Time=SimPar.Fail.Props.StopTime  After=-1  SampleTime=0
  Subsystem : Subsystem
  Sum : Sum  Inputs=|++
  Terminator1 : Terminator
  PropAct : Outport
  wires:
  [EngPwr] -> Terminator1/1
  [EngAccel] -> Bus Creator/2  "EngAccel"
  Bus Creator/1 -> [Prop]
  First Order Dynamic Rate and Position Limited Servo/2 -> [EngAccel]
  [Prop] -> PropAct/1
  [EngSpeed] -> Bus Creator/1  "EngSpeed"
  EngPwr/1 -> [EngPwr]
  EngCmd/1 -> [EngCmd]
  [EngCmd] -> First Order Dynamic Rate and Position Limited Servo/1
  First Order Dynamic Rate and Position Limited Servo/1 -> [EngSpeed]
  F_Up_Rlim/1 -> Subsystem/10(Up_Rlim)  "F_Up_Rlim"
  Subsystem/4(O_Pos_Bias) -> Bus Creator1/5  "F_Pos_Bias"
  F_Accel_Bias/1 -> Subsystem/12(Accel_Bias)  "F_Accel_Bias"
  Subsystem/11(O_Lwr_Rlim) -> Bus Creator1/12  "F_Lwr_Rlim"
  F_Pos_Bias/1 -> Subsystem/4(Pos_Bias)  "F_Pos_Bias"
  F_Rate_Bias/1 -> Subsystem/8(Rate_Bias)  "F_Rate_Bias"
  Constant2/1 -> Subsystem/17(MinPos)  "MinPos"
  F_Up_Alim/1 -> Subsystem/14(Up_Alim)  "F_Up_Alim"
  Product/1 -> Subsystem/1(Fail_Init), Bus Creator1/1  "F_Fail_Initiate"
  F_Pre_Scale/1 -> Subsystem/2(Pre_Scale)  "F_Pre_Scale"
  F_Pos_Scale/1 -> Subsystem/5(Pos_Scale)  "F_Pos_Scale"
  F_Fail_Initiate/1 -> Product/2  "F_Fail_Initiate"
  Subsystem/13(O_Accel_Scale) -> Bus Creator1/14  "F_Accel_Scale"
  F_Rate_Scale/1 -> Subsystem/9(Rate_Scale)  "F_Rate_Scale"
  Constant1/1 -> Subsystem/18(MaxRate)  "MaxRate"
  F_Lwr_Rlim/1 -> Subsystem/11(Lwr_Rlim)  "F_Lwr_Rlim"
  F_Lwr_Plim/1 -> Subsystem/7(Lwr_Plim)  "F_Lwr_Plim"
  Subsystem/12(O_Accel_Bias) -> Bus Creator1/13  "F_Accel_Bias"
  Constant3/1 -> Subsystem/19(MinRate)  "MinRate"
  Subsystem/5(O_Pos_Scale) -> Bus Creator1/6  "F_Pos_Scale"
  Subsystem/2(O_Pre_Scale) -> Bus Creator1/3  "F_Pre_Scale"
  Subsystem/7(O_Lwr_Plim) -> Bus Creator1/8  "F_Lwr_Plim"
  F_Accel_Scale/1 -> Subsystem/13(Accel_Scale)  "F_Accel_Scale"
  F_Post_Scale/1 -> Subsystem/3(Post_Scale)  "F_Post_Scale"
  Subsystem/14(O_Up_Alim) -> Bus Creator1/15  "F_Up_Alim"
  F_Lwr_Alim/1 -> Subsystem/15(Lwr_Alim)  "F_Lwr_Alim"
  Step/1 -> Sum/1
  Subsystem/10(O_Up_Rlim) -> Bus Creator1/11  "F_Up_Rlim"
  Bus Creator1/1 -> [Failure_Props]
  Subsystem/6(O_Up_Plim) -> Bus Creator1/7  "F_Up_Plim"
  Subsystem/8(O_Rate_Bias) -> Bus Creator1/9  "F_Rate_Bias"
  Constant4/1 -> Bus Creator1/17, Subsystem/20(Gen_Sig_Sel)  "F_Gen_Sig_Sel"
  F_Up_Plim/1 -> Subsystem/6(Up_Plim)  "F_Up_Plim"
  Step1/1 -> Sum/2
  Subsystem/15(O_Lwr_Alim) -> Bus Creator1/16  "F_Lwr_Alim"
  Constant/1 -> Subsystem/16(MaxPos)  "MaxPos"
  Subsystem/1(O_Hold_Last) -> Bus Creator1/2  "F_Hold_Last"
  Sum/1 -> Product/1
  Subsystem/3(O_Post_Scale) -> Bus Creator1/4  "F_Post_Scale"
  Subsystem/9(O_Rate_Scale) -> Bus Creator1/10  "F_Rate_Scale"
  [Failure_Props] -> First Order Dynamic Rate and Position Limited Servo/2
  [Failure_Props] -> Bus Creator/3  "Failure"

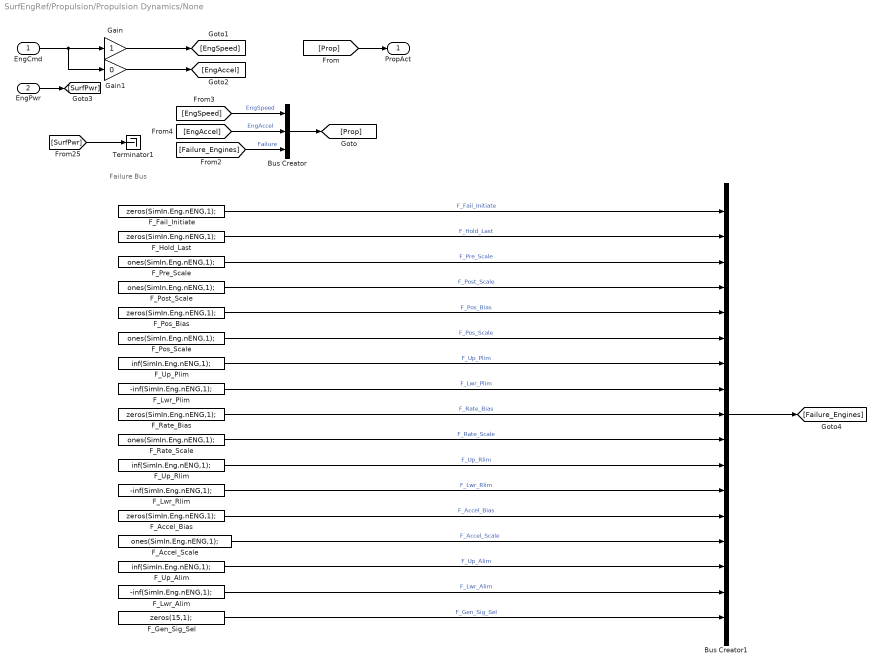
== system SurfEngRef/Propulsion/Propulsion Dynamics/None ==
  note: Failure Bus
  EngCmd : Inport
  EngPwr : Inport  Port=2
  Bus Creator : BusCreator  Inputs=3  OutDataTypeStr=Bus: BUS_PROP_ACTUATOR
  Bus Creator1 : BusCreator  Inputs=17  OutDataTypeStr=Bus: BUS_FAILURE_ENG
  F_Accel_Bias : Constant  Value=zeros(SimIn.Eng.nENG,1);
  F_Accel_Scale : Constant  Value=ones(SimIn.Eng.nENG,1);
  F_Fail_Initiate : Constant  Value=zeros(SimIn.Eng.nENG,1);
  F_Gen_Sig_Sel : Constant  Value=zeros(15,1);
  F_Hold_Last : Constant  Value=zeros(SimIn.Eng.nENG,1);
  F_Lwr_Alim : Constant  Value=-inf(SimIn.Eng.nENG,1);
  F_Lwr_Plim : Constant  Value=-inf(SimIn.Eng.nENG,1);
  F_Lwr_Rlim : Constant  Value=-inf(SimIn.Eng.nENG,1);
  F_Pos_Bias : Constant  Value=zeros(SimIn.Eng.nENG,1);
  F_Pos_Scale : Constant  Value=ones(SimIn.Eng.nENG,1);
  F_Post_Scale : Constant  Value=ones(SimIn.Eng.nENG,1);
  F_Pre_Scale : Constant  Value=ones(SimIn.Eng.nENG,1);
  F_Rate_Bias : Constant  Value=zeros(SimIn.Eng.nENG,1);
  F_Rate_Scale : Constant  Value=ones(SimIn.Eng.nENG,1);
  F_Up_Alim : Constant  Value=inf(SimIn.Eng.nENG,1);
  F_Up_Plim : Constant  Value=inf(SimIn.Eng.nENG,1);
  F_Up_Rlim : Constant  Value=inf(SimIn.Eng.nENG,1);
  Gain : Gain
  Gain1 : Gain  Gain=0
  Terminator1 : Terminator
  PropAct : Outport
  wires:
  [Failure_Engines] -> Bus Creator/3  "Failure"
  F_Fail_Initiate/1 -> Bus Creator1/1  "F_Fail_Initiate"
  Bus Creator1/1 -> [Failure_Engines]
  F_Rate_Scale/1 -> Bus Creator1/10  "F_Rate_Scale"
  F_Up_Rlim/1 -> Bus Creator1/11  "F_Up_Rlim"
  F_Lwr_Plim/1 -> Bus Creator1/8  "F_Lwr_Plim"
  F_Pre_Scale/1 -> Bus Creator1/3  "F_Pre_Scale"
  F_Pos_Scale/1 -> Bus Creator1/6  "F_Pos_Scale"
  F_Rate_Bias/1 -> Bus Creator1/9  "F_Rate_Bias"
  F_Accel_Bias/1 -> Bus Creator1/13  "F_Accel_Bias"
  F_Hold_Last/1 -> Bus Creator1/2  "F_Hold_Last"
  F_Lwr_Rlim/1 -> Bus Creator1/12  "F_Lwr_Rlim"
  F_Lwr_Alim/1 -> Bus Creator1/16  "F_Lwr_Alim"
  F_Post_Scale/1 -> Bus Creator1/4  "F_Post_Scale"
  F_Accel_Scale/1 -> Bus Creator1/14  "F_Accel_Scale"
  F_Pos_Bias/1 -> Bus Creator1/5  "F_Pos_Bias"
  F_Up_Plim/1 -> Bus Creator1/7  "F_Up_Plim"
  F_Up_Alim/1 -> Bus Creator1/15  "F_Up_Alim"
  F_Gen_Sig_Sel/1 -> Bus Creator1/17  "F_Gen_Sig_Sel"
  Gain1/1 -> [EngAccel]
  [Prop] -> PropAct/1
  [EngAccel] -> Bus Creator/2  "EngAccel"
  [EngSpeed] -> Bus Creator/1  "EngSpeed"
  [SurfPwr] -> Terminator1/1
  EngPwr/1 -> [SurfPwr]
  EngCmd/1 -> Gain/1, Gain1/1
  Bus Creator/1 -> [Prop]
  Gain/1 -> [EngSpeed]

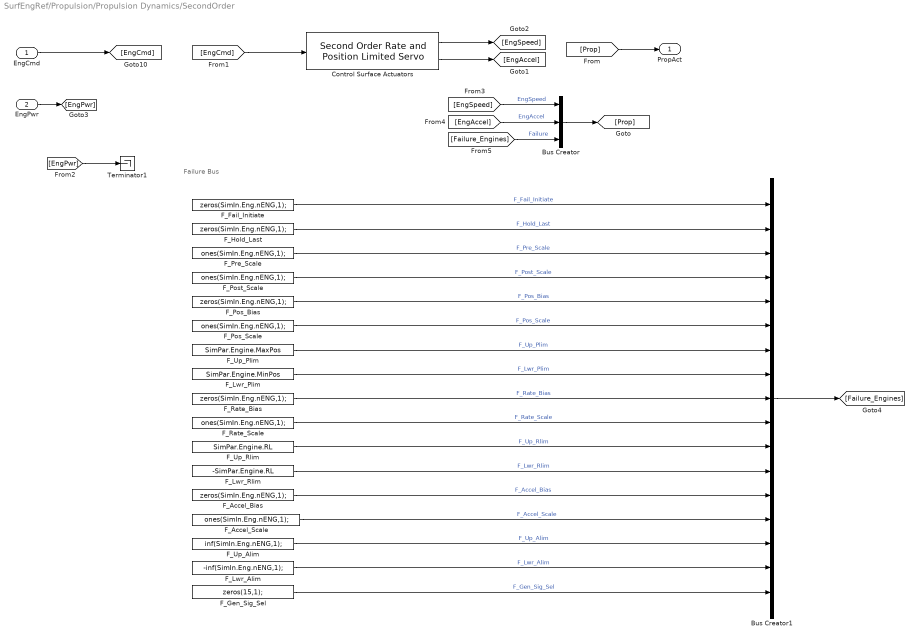
== system SurfEngRef/Propulsion/Propulsion Dynamics/SecondOrder ==
  note: Failure Bus
  EngCmd : Inport
  EngPwr : Inport  Port=2
  Bus Creator : BusCreator  Inputs=3  OutDataTypeStr=Bus: BUS_PROP_ACTUATOR
  Bus Creator1 : BusCreator  Inputs=17  OutDataTypeStr=Bus: BUS_FAILURE_ENG
  Control Surface Actuators : ServosLib/Second Order Rate and Position Limited Servo  freq=SimPar.Engine.BW  zeta=SimPar.Engine.Zeta  RL=SimPar.Engine.RL  POS_hi=SimPar.Engine.MaxPos  POS_lo=SimPar.Engine.MinPos  Bias=SimPar.Engine.Bias  PosStateName=EngineSpeed  RateStateName=EngineAccel
  F_Accel_Bias : Constant  Value=zeros(SimIn.Eng.nENG,1);
  F_Accel_Scale : Constant  Value=ones(SimIn.Eng.nENG,1);
  F_Fail_Initiate : Constant  Value=zeros(SimIn.Eng.nENG,1);
  F_Gen_Sig_Sel : Constant  Value=zeros(15,1);
  F_Hold_Last : Constant  Value=zeros(SimIn.Eng.nENG,1);
  F_Lwr_Alim : Constant  Value=-inf(SimIn.Eng.nENG,1);
  F_Lwr_Plim : Constant  Value=SimPar.Engine.MinPos
  F_Lwr_Rlim : Constant  Value=-SimPar.Engine.RL
  F_Pos_Bias : Constant  Value=zeros(SimIn.Eng.nENG,1);
  F_Pos_Scale : Constant  Value=ones(SimIn.Eng.nENG,1);
  F_Post_Scale : Constant  Value=ones(SimIn.Eng.nENG,1);
  F_Pre_Scale : Constant  Value=ones(SimIn.Eng.nENG,1);
  F_Rate_Bias : Constant  Value=zeros(SimIn.Eng.nENG,1);
  F_Rate_Scale : Constant  Value=ones(SimIn.Eng.nENG,1);
  F_Up_Alim : Constant  Value=inf(SimIn.Eng.nENG,1);
  F_Up_Plim : Constant  Value=SimPar.Engine.MaxPos
  F_Up_Rlim : Constant  Value=SimPar.Engine.RL
  Terminator1 : Terminator
  PropAct : Outport
  wires:
  [Failure_Engines] -> Bus Creator/3  "Failure"
  F_Up_Alim/1 -> Bus Creator1/15  "F_Up_Alim"
  F_Pos_Scale/1 -> Bus Creator1/6  "F_Pos_Scale"
  F_Fail_Initiate/1 -> Bus Creator1/1  "F_Fail_Initiate"
  Bus Creator1/1 -> [Failure_Engines]
  F_Pos_Bias/1 -> Bus Creator1/5  "F_Pos_Bias"
  F_Hold_Last/1 -> Bus Creator1/2  "F_Hold_Last"
  F_Up_Plim/1 -> Bus Creator1/7  "F_Up_Plim"
  F_Pre_Scale/1 -> Bus Creator1/3  "F_Pre_Scale"
  F_Gen_Sig_Sel/1 -> Bus Creator1/17  "F_Gen_Sig_Sel"
  F_Accel_Bias/1 -> Bus Creator1/13  "F_Accel_Bias"
  F_Lwr_Plim/1 -> Bus Creator1/8  "F_Lwr_Plim"
  F_Accel_Scale/1 -> Bus Creator1/14  "F_Accel_Scale"
  F_Up_Rlim/1 -> Bus Creator1/11  "F_Up_Rlim"
  F_Post_Scale/1 -> Bus Creator1/4  "F_Post_Scale"
  F_Rate_Bias/1 -> Bus Creator1/9  "F_Rate_Bias"
  F_Lwr_Rlim/1 -> Bus Creator1/12  "F_Lwr_Rlim"
  F_Rate_Scale/1 -> Bus Creator1/10  "F_Rate_Scale"
  F_Lwr_Alim/1 -> Bus Creator1/16  "F_Lwr_Alim"
  EngPwr/1 -> [EngPwr]
  [Prop] -> PropAct/1
  [EngCmd] -> Control Surface Actuators/1
  EngCmd/1 -> [EngCmd]
  [EngPwr] -> Terminator1/1
  Control Surface Actuators/1 -> [EngSpeed]
  Control Surface Actuators/2 -> [EngAccel]
  Bus Creator/1 -> [Prop]
  [EngSpeed] -> Bus Creator/1  "EngSpeed"
  [EngAccel] -> Bus Creator/2  "EngAccel"

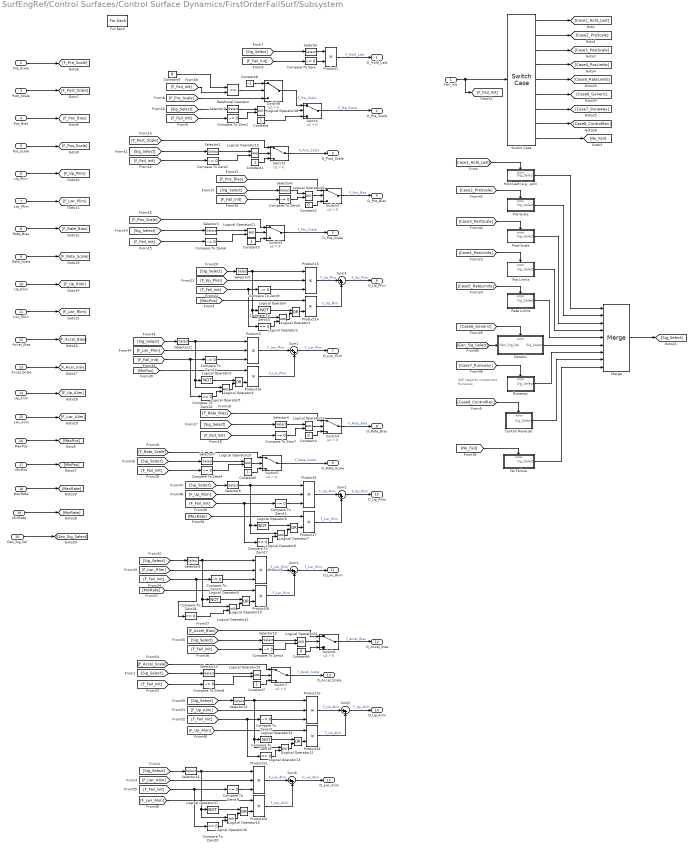
== system SurfEngRef/Control Surfaces/Control Surface Dynamics/FirstOrderFailSurf/Subsystem ==
  note: Still Need to Implement
      | Runaway
  Fail_Init : Inport  Partition=on  PartitionDimension=1  PartitionWidth=1  PartitionOffset=0
  Pre_Scale : Inport  Port=2  Partition=on  PartitionDimension=1  PartitionWidth=1  PartitionOffset=0
  Post_Scale : Inport  Port=3  Partition=on  PartitionDimension=1  PartitionWidth=1  PartitionOffset=0
  Pos_Bias : Inport  Port=4  Partition=on  PartitionDimension=1  PartitionWidth=1  PartitionOffset=0
  Pos_Scale : Inport  Port=5  Partition=on  PartitionDimension=1  PartitionWidth=1  PartitionOffset=0
  Up_Plim : Inport  Port=6  Partition=on  PartitionDimension=1  PartitionWidth=1  PartitionOffset=0
  Lwr_Plim : Inport  Port=7  Partition=on  PartitionDimension=1  PartitionWidth=1  PartitionOffset=0
  Rate_Bias : Inport  Port=8  Partition=on  PartitionDimension=1  PartitionWidth=1  PartitionOffset=0
  Rate_Scale : Inport  Port=9  Partition=on  PartitionDimension=1  PartitionWidth=1  PartitionOffset=0
  Up_Rlim : Inport  Port=10  Partition=on  PartitionDimension=1  PartitionWidth=1  PartitionOffset=0
  Lwr_Rlim : Inport  Port=11  Partition=on  PartitionDimension=1  PartitionWidth=1  PartitionOffset=0
  Accel_Bias : Inport  Port=12  Partition=on  PartitionDimension=1  PartitionWidth=1  PartitionOffset=0
  Accel_Scale : Inport  Port=13  Partition=on  PartitionDimension=1  PartitionWidth=1  PartitionOffset=0
  Up_Alim : Inport  Port=14  Partition=on  PartitionDimension=1  PartitionWidth=1  PartitionOffset=0
  Lwr_Alim : Inport  Port=15  Partition=on  PartitionDimension=1  PartitionWidth=1  PartitionOffset=0
  MaxPos : Inport  Port=16  Partition=on  PartitionDimension=1  PartitionWidth=1  PartitionOffset=0
  MinPos : Inport  Port=17  Partition=on  PartitionDimension=1  PartitionWidth=1  PartitionOffset=0
  MaxRate : Inport  Port=18  Partition=on  PartitionDimension=1  PartitionWidth=1  PartitionOffset=0
  MinRate : Inport  Port=19  Partition=on  PartitionDimension=1  PartitionWidth=1  PartitionOffset=0
  Gen_Sig_Sel : Inport  Port=20
  Compare To Zero{,1..14} (15 alike) : simulink/Logic and Bit Operations/Compare To Zero  relop=~=  OutDataTypeStr=boolean
  Compare To Zero{15..20} (6 alike) : simulink/Logic and Bit Operations/Compare To Zero  relop===  OutDataTypeStr=boolean
  Constant{,1,3,5,7} (5 alike) : Constant
  Constant2 : Constant  Value=0
  Constant4 : Constant  Value=0
  Constant6 : Constant  Value=0
  Constant8 : Constant  Value=-1
  Constant9 : Constant  Value=8
  Control Reversal : Subsystem  TreatAsAtomicUnit=on
  For Each : ForEach  DisableCoverage=on
  Generic : Subsystem  TreatAsAtomicUnit=on
  "Hold Last (e.g., jam)" : Subsystem  TreatAsAtomicUnit=on
  Logical Operator{,3,6,9,14,17} (6 alike) : Logic  Operator=NOT  AllPortsSameDT=off  OutDataTypeStr=boolean
  Logical Operator{1,4,7,10,12,15} (6 alike) : Logic  Operator=OR  AllPortsSameDT=off  OutDataTypeStr=boolean
  Logical Operator{2,5,8,11,13,16,18..25} (14 alike) : Logic  AllPortsSameDT=off  OutDataTypeStr=boolean
  Merge : Merge  Inputs=9  InitialOutput=7
  No Failure : Subsystem  TreatAsAtomicUnit=on
  Pos Limits : Subsystem  TreatAsAtomicUnit=on
  Post-Scale : Subsystem  TreatAsAtomicUnit=on
  Pre-Scale : Subsystem  TreatAsAtomicUnit=on
  Product{1,14,16..20} (7 alike) : Product
  Product{3..4,6,10,12,15} (6 alike) : Product  Inputs=3
  Rate Limits : Subsystem  TreatAsAtomicUnit=on
  Relational Operator : RelationalOperator  Operator===  OutDataTypeStr=boolean  RndMeth=Simplest  InputSameDT=off
  Runaway : Subsystem  TreatAsAtomicUnit=on
  Selector : Selector  IndexOptions=Index vector (dialog)  Indices=1  OutputSizes=1
  Selector1 : Selector  IndexOptions=Index vector (dialog)  Indices=2  OutputSizes=1
  Selector10 : Selector  IndexOptions=Index vector (dialog)  Indices=12  OutputSizes=1
  Selector11 : Selector  IndexOptions=Index vector (dialog)  Indices=7  OutputSizes=1
  Selector12 : Selector  IndexOptions=Index vector (dialog)  Indices=14  OutputSizes=1
  Selector13 : Selector  IndexOptions=Index vector (dialog)  Indices=13  OutputSizes=1
  Selector14 : Selector  IndexOptions=Index vector (dialog)  Indices=15  OutputSizes=1
  Selector2 : Selector  IndexOptions=Index vector (dialog)  Indices=3  OutputSizes=1
  Selector3 : Selector  IndexOptions=Index vector (dialog)  Indices=5  OutputSizes=1
  Selector4 : Selector  IndexOptions=Index vector (dialog)  Indices=8  OutputSizes=1
  Selector5 : Selector  IndexOptions=Index vector (dialog)  Indices=6  OutputSizes=1
  Selector6 : Selector  IndexOptions=Index vector (dialog)  Indices=4  OutputSizes=1
  Selector7 : Selector  IndexOptions=Index vector (dialog)  Indices=9  OutputSizes=1
  Selector8 : Selector  IndexOptions=Index vector (dialog)  Indices=10  OutputSizes=1
  Selector9 : Selector  IndexOptions=Index vector (dialog)  Indices=11  OutputSizes=1
  Sum{1..6} (6 alike) : Sum  Inputs=|++
  Switch{,1..8} (9 alike) : Switch  Criteria=u2 > Threshold  SaturateOnIntegerOverflow=off  InputSameDT=off
  Switch Case : SwitchCase  CaseConditions={1, 2, 3, 4, 5, 6, 7, 8}
  O_Hold_Last : Outport  ConcatenationDimension=1
  O_Pre_Scale : Outport  Port=2  ConcatenationDimension=1
  O_Post_Scale : Outport  Port=3  ConcatenationDimension=1
  O_Pos_Bias : Outport  Port=4  ConcatenationDimension=1
  O_Pos_Scale : Outport  Port=5  ConcatenationDimension=1
  O_Up_Plim : Outport  Port=6  ConcatenationDimension=1
  O_Lwr_Plim : Outport  Port=7  ConcatenationDimension=1
  O_Rate_Bias : Outport  Port=8  ConcatenationDimension=1
  O_Rate_Scale : Outport  Port=9  ConcatenationDimension=1
  O_Up_Rlim : Outport  Port=10  ConcatenationDimension=1
  O_Lwr_Rlim : Outport  Port=11  ConcatenationDimension=1
  O_Accel_Bias : Outport  Port=12  ConcatenationDimension=1
  O_Accel_Scale : Outport  Port=13  ConcatenationDimension=1
  O_Up_Alim : Outport  Port=14  ConcatenationDimension=1
  O_Lwr_Alim : Outport  Port=15  ConcatenationDimension=1
  wires:
  Gen_Sig_Sel/1 -> [Gen_Sig_Select]
  [Gen_Sig_Select] -> Generic/1(Gen_Sig_Sel)
  Merge/1 -> [Sig_Select]
  Logical Operator2/1 -> Logical Operator1/2
  Compare To Zero15/1 -> Logical Operator2/2
  Logical Operator1/1 -> Product14/2
  Logical Operator/1 -> Logical Operator1/1
  [MaxPos] -> Product14/1
  Product14/1 -> Sum3/2  "F_Up_Plim"
  Product15/1 -> Sum3/1  "F_Up_Plim"
  MaxRate/1 -> [MaxRate]
  MinRate/1 -> [MinRate]
  MinPos/1 -> [MinPos]
  MaxPos/1 -> [MaxPos]
  [Sig_Select] -> Selector14/1
  [F_Lwr_Alim] -> Product12/2
  [F_Accel_Scale] -> Switch7/1
  [F_Fail_Init] -> Compare To Zero8/1
  Compare To Zero8/1 -> Logical Operator25/2
  Selector13/1 -> Logical Operator25/1
  [Sig_Select] -> Selector13/1
  Selector10/1 -> Logical Operator24/1
  [Sig_Select] -> Selector10/1
  [F_Fail_Init] -> Compare To Zero3/1
  Compare To Zero3/1 -> Logical Operator24/2
  [F_Up_Alim] -> Product10/2
  [Sig_Select] -> Selector12/1
  [F_Accel_Bias] -> Switch6/1
  [F_Lwr_Rlim] -> Product6/2
  [Sig_Select] -> Selector9/1
  [F_Fail_Init] -> Compare To Zero17/1, Compare To Zero11/1
  [Sig_Select] -> Selector8/1
  Switch5/1 -> O_Rate_Scale/1  "F_Rate_Scale"
  [F_Rate_Scale] -> Switch5/1
  Compare To Zero4/1 -> Logical Operator23/2
  [Sig_Select] -> Selector7/1
  Selector7/1 -> Logical Operator23/1
  [F_Fail_Init] -> Compare To Zero4/1
  Switch4/1 -> O_Rate_Bias/1  "F_Rate_Bias"
  [F_Rate_Bias] -> Switch4/1
  Selector4/1 -> Logical Operator22/1
  [Sig_Select] -> Selector4/1
  Compare To Zero7/1 -> Logical Operator22/2
  [F_Fail_Init] -> Compare To Zero7/1
  [F_Fail_Init] -> Compare To Zero6/1
  Compare To Zero6/1 -> Logical Operator21/2
  [Sig_Select] -> Selector3/1
  Selector3/1 -> Logical Operator21/1
  [F_Pos_Scale] -> Switch3/1
  Switch2/1 -> O_Pos_Bias/1  "F_Pos_Bias"
  [Sig_Select] -> Selector6/1
  Selector6/1 -> Logical Operator20/1
  Compare To Zero5/1 -> Logical Operator20/2
  [F_Fail_Init] -> Compare To Zero5/1
  [F_Pos_Bias] -> Switch2/1
  Compare To Zero2/1 -> Logical Operator19/2
  Compare To Zero1/1 -> Logical Operator18/2
  Generic/1(Sig_Select) -> Merge/6
  Runaway/1(Sig_Select) -> Merge/7
  [Case7_Runaway] -> Runaway/Action
  [Case6_Generic] -> Generic/Action
  No Failure/1(Sig_Select) -> Merge/9
  [No_Fail] -> No Failure/Action
  Switch6/1 -> O_Accel_Bias/1  "F_Accel_Bias"
  "Hold Last (e.g., jam)"/1(Sig_Select) -> Merge/1
  Product6/1 -> Sum4/1  "F_Lwr_Rlim"
  Product4/1 -> Sum2/1  "F_Up_Rlim"
  Product3/1 -> Sum1/1  "F_Lwr_Plim"
  Selector5/1 -> Product15/1, Logical Operator/1, Logical Operator2/1
  [Sig_Select] -> Selector5/1
  [F_Up_Plim] -> Product15/2
  Sum3/1 -> O_Up_Plim/1  "F_Up_Plim"
  Switch3/1 -> O_Pos_Scale/1  "F_Pos_Scale"
  Switch1/1 -> O_Post_Scale/1  "F_Post_Scale"
  Selector1/1 -> Logical Operator18/1
  [Sig_Select] -> Selector1/1
  [F_Pre_Scale] -> Switch8/3
  Switch/1 -> O_Pre_Scale/1  "F_Pre_Scale"
  [Sig_Select] -> Selector/1
  Product1/1 -> O_Hold_Last/1  "F_Hold_Last"
  Selector/1 -> Product1/1
  Product12/1 -> Sum6/1  "F_Lwr_Alim"
  Switch7/1 -> O_Accel_Scale/1  "F_Accel_Scale"
  Lwr_Alim/1 -> [F_Lwr_Alim]
  Up_Alim/1 -> [F_Up_Alim]
  Accel_Scale/1 -> [F_Accel_Scale]
  Accel_Bias/1 -> [F_Accel_Bias]
  Lwr_Rlim/1 -> [F_Lwr_Rlim]
  Up_Rlim/1 -> [F_Up_Rlim]
  Rate_Scale/1 -> [F_Rate_Scale]
  Rate_Bias/1 -> [F_Rate_Bias]
  Lwr_Plim/1 -> [F_Lwr_Plim]
  Up_Plim/1 -> [F_Up_Plim]
  Pos_Scale/1 -> [F_Pos_Scale]
  Pos_Bias/1 -> [F_Pos_Bias]
  Post_Scale/1 -> [F_Post_Scale]
  Pre_Scale/1 -> [F_Pre_Scale]
  Switch Case/9 -> [No_Fail]
  [Case1_Hold_Last] -> "Hold Last (e.g., jam)"/Action
  Switch Case/1 -> [Case1_Hold_Last]
  Fail_Init/1 -> [F_Fail_Init], Switch Case/1
  Switch Case/2 -> [Case2_PreScale]
  Switch Case/3 -> [Case3_PostScale]
  Switch Case/4 -> [Case4_PosLimits]
  Switch Case/5 -> [Case5_RateLimits]
  Switch Case/6 -> [Case6_Generic]
  Switch Case/7 -> [Case7_Runaway]
  Switch Case/8 -> [Case8_ControlRev]
  [Case8_ControlRev] -> Control Reversal/Action
  Control Reversal/1(Sig_Select) -> Merge/8
  [Case2_PreScale] -> Pre-Scale/Action
  Compare To Zero/1 -> Product1/2
  [F_Fail_Init] -> Compare To Zero/1
  [F_Fail_Init] -> Compare To Zero1/1
  [F_Fail_Init] -> Compare To Zero2/1
  [Sig_Select] -> Selector2/1
  Selector2/1 -> Logical Operator19/1
  [F_Post_Scale] -> Switch1/1
  Post-Scale/1(Sig_Select) -> Merge/3
  [Case3_PostScale] -> Post-Scale/Action
  Pre-Scale/1(Sig_Select) -> Merge/2
  [F_Fail_Init] -> Compare To Zero9/1, Compare To Zero15/1
  [F_Fail_Init] -> Compare To Zero16/1, Compare To Zero10/1
  [Sig_Select] -> Selector11/1
  [Case4_PosLimits] -> Pos Limits/Action
  Pos Limits/1(Sig_Select) -> Merge/4
  [Case5_RateLimits] -> Rate Limits/Action
  Rate Limits/1(Sig_Select) -> Merge/5
  [F_Lwr_Plim] -> Product3/2
  [F_Up_Rlim] -> Product4/2
  Compare To Zero9/1 -> Product15/3
  Compare To Zero11/1 -> Product4/3
  Compare To Zero12/1 -> Product6/3
  Compare To Zero13/1 -> Product10/3
  Compare To Zero14/1 -> Product12/3
  Product10/1 -> Sum5/1  "F_Up_Alim"
  Compare To Zero10/1 -> Product3/3
  Selector11/1 -> Logical Operator3/1, Logical Operator5/1, Product3/1
  Logical Operator5/1 -> Logical Operator4/2
  Compare To Zero16/1 -> Logical Operator5/2
  Logical Operator3/1 -> Logical Operator4/1
  Logical Operator4/1 -> Product16/2
  [MinPos] -> Product16/1
  Product16/1 -> Sum1/2  "F_Lwr_Plim"
  Sum1/1 -> O_Lwr_Plim/1  "F_Lwr_Plim"
  Logical Operator7/1 -> Product17/2
  Logical Operator6/1 -> Logical Operator7/1
  Selector8/1 -> Logical Operator6/1, Logical Operator8/1, Product4/1
  Compare To Zero17/1 -> Logical Operator8/2
  Logical Operator8/1 -> Logical Operator7/2
  Sum2/1 -> O_Up_Rlim/1  "F_Up_Rlim"
  Product17/1 -> Sum2/2  "F_Lwr_Rlim"
  [MaxRate] -> Product17/1
  Compare To Zero18/1 -> Logical Operator11/2
  Product18/1 -> Sum4/2  "F_Lwr_Rlim"
  Logical Operator9/1 -> Logical Operator10/1
  Logical Operator10/1 -> Product18/2
  [F_Fail_Init] -> Compare To Zero18/1, Compare To Zero12/1
  Selector9/1 -> Logical Operator9/1, Logical Operator11/1, Product6/1
  Logical Operator11/1 -> Logical Operator10/2
  Sum4/1 -> O_Lwr_Rlim/1  "F_Lwr_Rlim"
  [MinRate] -> Product18/1
  Logical Operator13/1 -> Logical Operator12/2
  Logical Operator12/1 -> Product19/2
  Logical Operator14/1 -> Logical Operator12/1
  [F_Fail_Init] -> Compare To Zero19/1, Compare To Zero13/1
  Selector12/1 -> Logical Operator14/1, Logical Operator13/1, Product10/1
  Compare To Zero19/1 -> Logical Operator13/2
  Sum5/1 -> O_Up_Alim/1  "F_Up_Alim"
  [F_Up_Alim] -> Product19/1
  Selector14/1 -> Logical Operator17/1, Logical Operator16/1, Product12/1
  Logical Operator17/1 -> Logical Operator15/1
  Logical Operator16/1 -> Logical Operator15/2
  Compare To Zero20/1 -> Logical Operator16/2
  [F_Fail_Init] -> Compare To Zero20/1, Compare To Zero14/1
  Logical Operator15/1 -> Product20/2
  Sum6/1 -> O_Lwr_Alim/1  "F_Lwr_Alim"
  Product20/1 -> Sum6/2  "F_Lwr_Alim"
  [F_Lwr_Alim] -> Product20/1
  Product19/1 -> Sum5/2  "F_Up_Alim"
  Logical Operator18/1 -> Switch/2
  Constant/1 -> Switch/3
  Logical Operator19/1 -> Switch1/2
  Constant1/1 -> Switch1/3
  Constant2/1 -> Switch2/3
  Logical Operator20/1 -> Switch2/2
  Constant3/1 -> Switch3/3
  Logical Operator21/1 -> Switch3/2
  Logical Operator22/1 -> Switch4/2
  Constant4/1 -> Switch4/3
  Logical Operator23/1 -> Switch5/2
  Constant5/1 -> Switch5/3
  Logical Operator24/1 -> Switch6/2
  Constant6/1 -> Switch6/3
  Logical Operator25/1 -> Switch7/2
  Constant7/1 -> Switch7/3
  Switch8/1 -> Switch/1  "F_Pre_Scale"
  Constant8/1 -> Switch8/1
  [F_Fail_Init] -> Relational Operator/2
  Relational Operator/1 -> Switch8/2
  Constant9/1 -> Relational Operator/1
